simulink model "xNeuralSim_603"  (R2012b)
settings: Solver=FixedStepDiscrete  StartTime=0  StopTime=Inf  FixedStep=.0005  RelTol=1e-3
values from neighbouring files (symbols this model uses):
  cbhwlib_ver_major = 3    [buildXNeuralSim.m]    (also in xNeuralSim_Init.m)
  cbhwlib_ver_minor = 10    [buildXNeuralSim.m]    (also in xNeuralSim_Init.m = 9)
  enableNeuralSim = 1    [xNeuralSim_Init.m]
  max_num_cbpkts = 5    [xNeuralSim_Init.m]
  nch = 192    [xNeuralSim_Init.m]
  nsp_recv_port = 1001    [xNeuralSim_Init.m]
  nsp_send_port = 1002    [xNeuralSim_Init.m]
  sampleSendEnable_NSP1 = 1    [xNeuralSim_Init.m]
  sampleSendEnable_NSP2 = 1    [xNeuralSim_Init.m]
  spikeSendEnable_NSP1 = 1    [xNeuralSim_Init.m]
  spikeSendEnable_NSP2 = 1    [xNeuralSim_Init.m]
  unitMap = unitMap./repmat(sqrt(sum(unitMap.^2)), dimensions, 1)    [xNeuralSim_Init.m]
undefined symbols (not defined in the file or in its folder): macaddr
undefined symbols (not defined in the file): nsp1_pci_bus, nsp1_pci_slot
libraries: xpcethernetlib x15, xpcrtudplib x8, dspmtrx3 x7, xpclib x6, simulink x4, dspsrcs4 x2, xpciplib x2, xpcparallelportlib x1
(part 1 of 2)
settings Model: xpc_rtwmakecfg_data=_xpcetherlib__xpcether8255xlib__xpcetherGbElib__xpciplib__xpcnblib_  SimulationMode=external  TunableVars=enableNeuralSim  TunableVarsStorageClass=Auto  Creator=operator  LastModifiedBy=NPTL
settings SolverCC: EnableConcurrentExecution=on  InsertRTBMode=Always
settings DataIOCC: SignalLoggingSaveFormat=ModelDataLogs  DSMLogging=off
settings OptimizationCC: BlockReduction=off  InlineParams=on  InlineInvariantSignals=on  EnhancedBackFolding=on  EfficientFloat2IntCast=on  SimCompilerOptimization=On  AccelVerboseBuild=on
settings DebuggingCC: InheritedTsInSrcMsg=none  FcnCallInpInsideContextMsg=UseLocalSettings
settings HardwareCC: ProdIntDivRoundTo=Zero  ProdEndianess=LittleEndian  ProdHWDeviceType=Generic->32-bit x86 compatible
settings ModelReferenceCC: UpdateModelReferenceTargets=Force  EnableParallelModelReferenceBuilds=on
settings SFSimCC: SimBuildMode=sf_make_clean
settings RTWCC: SystemTargetFile=xpctarget.tlc  TLCOptions=-axPCMaxOverloads=100000  TemplateMakefile=xpc_default_tmf  Description=xPC Target  ProcessScript=xpctarget_make_rtw_hook  RTWCompilerOptimization=On
settings xpcTargetCC: TargetFcnLib=ansi_tfl_table_tmw.mat  CodeReplacementLibrary=XPC_BLAS  ParMdlRefBuildCompliant=on  ConcurrentExecutionCompliant=on  CombineSignalStateStructs=off  GRTInterface=on  RL32LogBufSizeModifier=10000  xPCTaskExecutionProfile=off  xPCRL32EventNumber=5000  RL32ObjectName=tgs  xPCisDefaultEnv=off  xPCTargetPCEnvName=xSimTarget  xPCLoadParamSetFile=off  xPCConcurrentTasks=on  xPCEnableSFAnimation=off

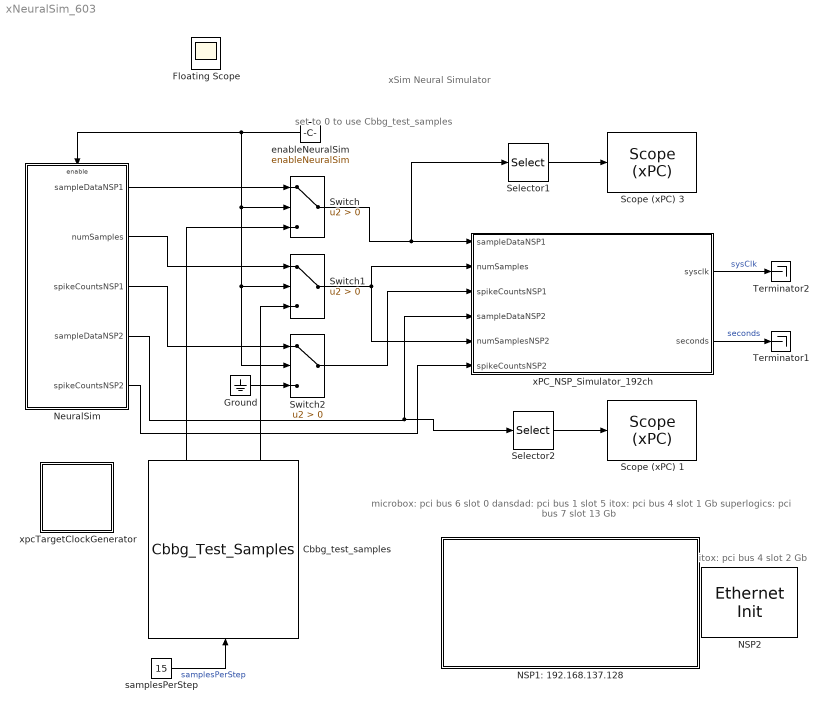
== system xNeuralSim_603 ==
  note: set to 0 to use
      | Cbbg_test_samples
  note: microbox: pci bus 6 slot 0
      | dansdad: pci bus 1 slot 5
      | itox: pci bus 4 slot 1 Gb
      | superlogics: pci bus 7 slot 13 Gb
  note: itox: pci bus 4 slot 2 Gb
  note: xSim Neural Simulator
  Cbbg_test_samples : S-Function  InitFcn=try, set_param(gcb,'FunctionName','Cbbg_Test_Samples'), end  FunctionName=Cbbg_Test_Samples  SFunctionModules=Cbbg_Test_Samples_wrapper  EnableBusSupport=off  mask(S-Function Builder){}
      mask help: The S-Function Builder block creates a wrapper C-MEX S-function from your supplied C code with multiple input ports, output ports, and a variable number of scalar, vector, or matrix parameters. The input and output ports can propagate Simulink built-in data types, fixed-point datatypes, complex, frame, 1-D, and 2-D signals. This block also supports discrete and continuous states of type real. You can optionally have the block generate a TLC file to be used with Real-Time Workshop for code generation.
      mask init:
      | val = [[.9  0.75 0.75 1 1 .9 .9 1]',[1 1 0.75 0.75 .9 .9 1 .9]'];try , sys = get_param(gcb,'SfunBuilderFcnName');if isempty(sys), sys = get_param(gcb,'FunctionName'); end,catch, sys = get_param(gcb,'FunctionName'); end
      settings: CopyFcn=set_param(gcbh,'LinkStatus','none')  PreSaveFcn=try, set_param(gcb,'FunctionName','Cbbg_Test_Samples'), end  OpenFcn=sfunctionwizard(gcbh)
      mask Display: plot(val(:,1),val(:,2)),disp(sys), port_label('input',1,'samplesPerStep'), port_label('output',1,'sampleData'), port_label('output',2,'numSamples')
  Ground : Ground
  NSP1: 192.168.137.128 : Subsystem  mask(xpcnwconfig){IpAddress=192.168.137.128, SubnetMask=255.255.255.0, Gateway=0.0.0.0, EthDrv=Intel Gigabit, PciBus=nsp1_pci_bus, PciSlot=nsp1_pci_slot}
      mask prompts: IpAddress "IP Address:"; SubnetMask "Subnet Mask:"; EthDrv "Ethernet Driver"; PciBus "PCI Bus:"; PciSlot "PCI Slot:"
      mask help: Network Configuration
      mask init:
      | IpAddress = ipaddr(IpAddress);
      | SubnetMask = ipaddr(SubnetMask);
      | Gateway = ipaddr(Gateway);
      mask Help: eval('xpcdoc(''RT_NETWORK_CONFIGURATION'')');
      mask TypeOptions EthDrv: Intel 8255x | Intel Gigabit
      mask Display: image(imread('cerebus.png','png'));
  NSP2 : xpcethernetlib/Ethernet Init   ID=2  Driver=Intel Gigabit  Bus=nsp2_pci_bus  Slot=nsp2_pci_slot  SampleTime=-1  AddressSource=EEPROM  MAC=macaddr('2A:2B:3C:4D:5E:6F')  TxSA=off  RxPromiscuous=off  Multicast={}  RxBad=off  RxShort=off  MaxMTU=1518  TxThreshold=224  TxBuffers=8192  RxBuffers=8192  ShowTune=on  NumRxBlks=1
  NeuralSim : Subsystem
  Scope (xPC) 1 : xpclib/Misc./Scope (xPC)   scopeno=4  scopetype=Target  autostart=on  viewmode=Graphical sliding  formatstr='%15.6f'  grid=on  ylimits=[-600 600]  nosamples=1000  noprepostsamples=0  interleave=1  triggermode=FreeRun  triggersignal=1  triggerlevel=-400  triggerslope=Falling  triggerscope=1  triggersample=0  filename=data.dat  mode=Lazy  writesize=512  autorestart=off  dynamicfilemode=off  maxwritefilesize=512*1024^2
  Scope (xPC) 3 : xpclib/Misc./Scope (xPC)   scopeno=3  scopetype=Target  autostart=on  viewmode=Graphical sliding  formatstr='%15.6f'  grid=on  ylimits=[-600 600]  nosamples=1000  noprepostsamples=0  interleave=1  triggermode=FreeRun  triggersignal=1  triggerlevel=-400  triggerslope=Falling  triggerscope=1  triggersample=0  filename=data.dat  mode=Lazy  writesize=512  autorestart=off  dynamicfilemode=off  maxwritefilesize=512*1024^2
  Selector1 : Selector  IndexOptions=Index vector (dialog)  Indices=[1440]  OutputSizes=1
  Selector2 : Selector  IndexOptions=Index vector (dialog)  Indices=[1440]  OutputSizes=1
  Switch : Switch  Criteria=u2 > Threshold
  Switch1 : Switch  Criteria=u2 > Threshold
  Switch2 : Switch  Criteria=u2 > Threshold
  Terminator1 : Terminator
  Terminator2 : Terminator
  enableNeuralSim : Constant  Value=enableNeuralSim  OutDataTypeStr=Inherit: Inherit via back propagation
  samplesPerStep : Constant  Value=15  OutDataTypeStr=Inherit: Inherit via back propagation
  xPC_NSP_Simulator_192ch : Subsystem
  xpcTargetClockGenerator : Subsystem
  Floating Scope : Scope
      settings: Floating=on
  wires:
  xPC_NSP_Simulator_192ch/2(seconds) -> Terminator1/1  "seconds"
  NeuralSim/1(sampleDataNSP1) -> Switch/1
  NeuralSim/2(numSamples) -> Switch1/1
  NeuralSim/3(spikeCountsNSP1) -> Switch2/1
  Cbbg_test_samples/1 -> Switch/3
  Switch1/1 -> xPC_NSP_Simulator_192ch/5(numSamplesNSP2), xPC_NSP_Simulator_192ch/2(numSamples)
  Cbbg_test_samples/2 -> Switch1/3
  enableNeuralSim/1 -> NeuralSim/Enable, Switch2/2, Switch1/2, Switch/2
  samplesPerStep/1 -> Cbbg_test_samples/1  "samplesPerStep"
  xPC_NSP_Simulator_192ch/1(sysclk) -> Terminator2/1  "sysClk"
  Selector1/1 -> Scope (xPC) 3/1
  Switch2/1 -> xPC_NSP_Simulator_192ch/3(spikeCountsNSP1)
  Ground/1 -> Switch2/3
  Switch/1 -> Selector1/1, xPC_NSP_Simulator_192ch/1(sampleDataNSP1)
  NeuralSim/5(spikeCountsNSP2) -> xPC_NSP_Simulator_192ch/6(spikeCountsNSP2)
  Selector2/1 -> Scope (xPC) 1/1
  NeuralSim/4(sampleDataNSP2) -> Selector2/1, xPC_NSP_Simulator_192ch/4(sampleDataNSP2)

== system xNeuralSim_603/NSP1: 192.168.137.128 ==
  "ARP Init " : S-Function  Priority=0  FunctionName=xpcdebugarpinit  Parameters=Stats, Interface, IpAddress, SubnetMask, Gateway, EthernetId, Flags, BlockId, Retry, Timeout, Expiration, StaticAddressListIp, StaticAddressListMac, DiscoveryList, MulticastList, SampleTime  EnableBusSupport=off  mask(arpinit){Interface=0, IpAddress=IpAddress, SubnetMask=SubnetMask, Gateway=Gateway, EthernetId=1, BlockId=0, SampleTime=-1, Flags=hex2dec('00000697'), Stats=off, Retry=5, Timeout=20, Expiration=20*60, StaticAddressListIp=[], StaticAddressListMac=[], DiscoveryList=[], MulticastList=[]}
      mask prompts: IpAddress "IP Address"; SubnetMask "Subnet Mask"; EthernetId "Ethernet ID"; BlockId "Block ID"; SampleTime "Sample Time"; Stats "Statistics Port"; StaticAddressListIp "[Static IP]"; StaticAddressListMac "[Static MAC]"; DiscoveryList "[Discovery IP]"; MulticastList "[Multicast IP]"
      mask help: ARP Init
      mask init:
      | xpclinklib('xpciplib');
      mask Help: web('arpdebug.htm',  '-helpbrowser');
      mask Display: disp('ARP Init');
  "Buffer Mngmt " : S-Function  Priority=-1  FunctionName=xpcnb  Parameters=pool_sizes, SampleTime, ShowTune  EnableBusSupport=off  mask(xpcnbinit){SampleTime=-1, PoolSizes=[2048 2048 50000 50000], ShowTune=on}
      mask prompts: SampleTime "Sample time:"; PoolSizes "Buffer pool sizes (256, 512, 1024, 2048):"; ShowTune "Display tuning information"
      mask help: Network Buffer Initialization
      mask init:
      | [MaskDisplay, pool_sizes] = mxpcnbinit(2, PoolSizes);
      | 
      | set_param(gcb, 'MaskDisplay', MaskDisplay);
      mask Help: eval('xpcdoc(''NB_Init'')');
      mask Display: disp('Network Buffer\nManagement');
  "Ethernet Init " : S-Function  Priority=-1  FunctionName=xpcetherinit  Parameters="ID, Driver, Bus, Slot, VendorID, DeviceID, AddressSource, mac, TxSA, RxPromiscuous, RxBad, RxShort, MaxMTU, TxThreshold, TxBuffers, RxBuffers, ShowTune, numMulti, multicast,   NumRxBlks, SampleTime"  EnableBusSupport=off  mask(xpcetherinit){ID=1, Driver=EthDrv, Bus=PciBus, Slot=PciSlot, SampleTime=-1, AddressSource=EEPROM, MAC=macaddr('00:00:00:00:00:00'), TxSA=off, RxPromiscuous=off, Multicast={}, RxBad=off, RxShort=off, MaxMTU=1518, TxThreshold=224, TxBuffers=8192, RxBuffers=8192, ShowTune=on, NumRxBlks=1}
      mask prompts: ID "Device ID:"; Bus "PCI bus:"; Slot "PCI slot:"; SampleTime "Sample time:"; AddressSource "Address source:"; TxSA "Tx source address from model"; RxPromiscuous "Rx promiscuous"; Multicast "Multicast address list:"; RxBad "Rx bad frames"; RxShort "Rx short frames"; MaxMTU "Max MTU:"; TxThreshold "Tx threshold:"; TxBuffers "Tx buffers:"; RxBuffers "Rx buffers:"; ShowTune "Display tuning information"; NumRxBlks "num rx blocks"
      mask help: Ethernet Initialization
      mask init:
      | VendorID = -1;
      | DeviceID = -1;
      | 
      | [MaskDisplay, VendorID, DeviceID, mac, numMulti, multicast] = mxpcetherinit(2, ID, Driver, Bus, Slot, MAC, Multicast);
      | 
      | set_param(gcb, 'MaskDisplay', MaskDisplay);
      mask Help: eval('xpcdoc(''Ether_Init'')');
      mask TypeOptions ID: 1 | 2 | 3 | 4 | 5 | 6 | 7 | 8
      mask TypeOptions AddressSource: EEPROM | Specify
      mask Callback AddressSource:
      | enables = get_param(gcb, 'MaskVisibilities');
      | if strcmp('Specify', get_param(gcb, 'AddressSource'))
      |     enables{strmatch('MAC',fieldnames(get_param(gcb,'DialogParameters')))} = 'on';
      | else
      |     enables{strmatch('MAC',fieldnames(get_param(gcb,'DialogParameters')))} = 'off';
      | end
      | set_param(gcb, 'MaskVisibilities', enables);
      mask Display: disp('Ethernet\nInitialization\nbus: 4 slot: 0\nId: 1\nIntel Gigabit');
  "IP Init " : S-Function  Priority=1  FunctionName=xpcdebugipinit  Parameters=Stats, Group, ArpId, IpAddress, SubnetMask, DefaultGateway, DefaultInterface, Flags, ToS, StartingId, TTL, SampleTime  EnableBusSupport=off  mask(ipinit){Group=0, ArpId=[0], IpAddress=[IpAddress], SubnetMask=[SubnetMask], DefaultGateway=Gateway, DefaultInterface=0, SampleTime=-1, Flags=hex2dec('00000005'), ToS=hex2dec('00'), StartingId=10000, TTL=64, Stats=off}
      mask prompts: ArpId "[ARP ID]"; IpAddress "[IP Address]"; SubnetMask "[Subnet Mask]"; DefaultGateway "Default Gateway"; DefaultInterface "Default Interface"; SampleTime "Sample Time"; StartingId "Starting Id"; Stats "Statistics Port"
      mask help: IP Init
      mask init:
      | xpclinklib('xpciplib');
      mask Help: web('ipdebug.htm',  '-helpbrowser');
      mask Display: disp('IP Init');
  "UDP Init " : S-Function  Priority=2  FunctionName=xpcdebugudpinit  Parameters=Stats, Group, StartingPort, Flags, SampleTime  EnableBusSupport=off  mask(udpinit){Group=0, StartingPort=10000, Flags=hex2dec('00000001'), SampleTime=-1, Stats=off}
      mask prompts: StartingPort "Starting Port"; SampleTime "Sample Time"; Stats "Statistics Port"
      mask help: UDP Init
      mask init:
      | xpclinklib('xpciplib');
      mask Help: web('udpdebug.htm',  '-helpbrowser');
      mask Display: disp('UDP Init');

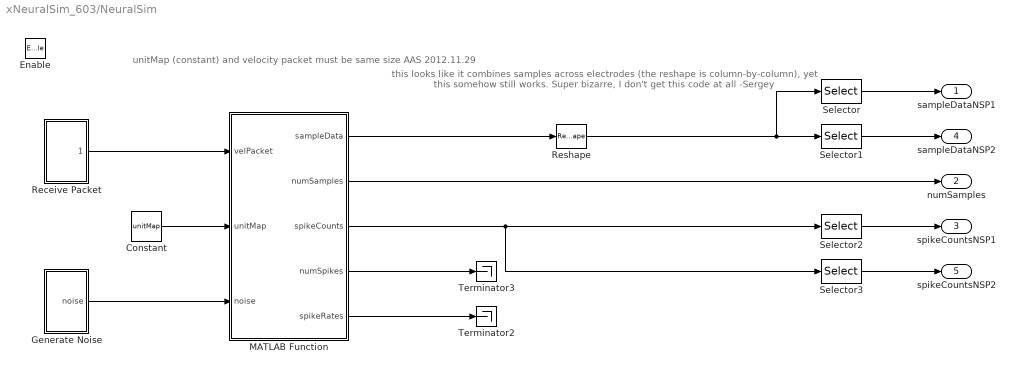
== system xNeuralSim_603/NeuralSim ==
  note: this looks like it combines samples across
      | electrodes (the reshape is column-by-column), yet this somehow still works.
      | Super bizarre, I don't get this code at all -Sergey
  note: unitMap (constant) and velocity
      | packet must be same size
      | AAS 2012.11.29
  Enable : EnablePort
  Constant : Constant  Value=unitMap
  Generate Noise : Subsystem
  MATLAB Function : MATLAB Function  TreatAsAtomicUnit=on
  Receive Packet : Subsystem
  Reshape : Reshape
  Selector : Selector  InputPortWidth=2880  IndexOptions=Starting index (dialog)  Indices=[1]  OutputSizes=1440
  Selector1 : Selector  InputPortWidth=2880  IndexOptions=Starting index (dialog)  Indices=[1441]  OutputSizes=1440
  Selector2 : Selector  InputPortWidth=192  IndexOptions=Starting index (dialog)  Indices=[1]  OutputSizes=96
  Selector3 : Selector  InputPortWidth=192  IndexOptions=Starting index (dialog)  Indices=[97]  OutputSizes=96
  Terminator2 : Terminator
  Terminator3 : Terminator
  sampleDataNSP1 : Outport
  numSamples : Outport  Port=2
  spikeCountsNSP1 : Outport  Port=3
  sampleDataNSP2 : Outport  Port=4
  spikeCountsNSP2 : Outport  Port=5
  wires:
  MATLAB Function/2(numSamples) -> numSamples/1
  MATLAB Function/4(numSpikes) -> Terminator3/1
  MATLAB Function/5(spikeRates) -> Terminator2/1
  Constant/1 -> MATLAB Function/2(unitMap)
  Receive Packet/1(velocity) -> MATLAB Function/1(velPacket)
  Generate Noise/1(noise) -> MATLAB Function/3(noise)
  Reshape/1 -> Selector/1, Selector1/1
  Selector/1 -> sampleDataNSP1/1
  Selector1/1 -> sampleDataNSP2/1
  Selector2/1 -> spikeCountsNSP1/1
  MATLAB Function/3(spikeCounts) -> Selector3/1, Selector2/1
  Selector3/1 -> spikeCountsNSP2/1
  MATLAB Function/1(sampleData) -> Reshape/1

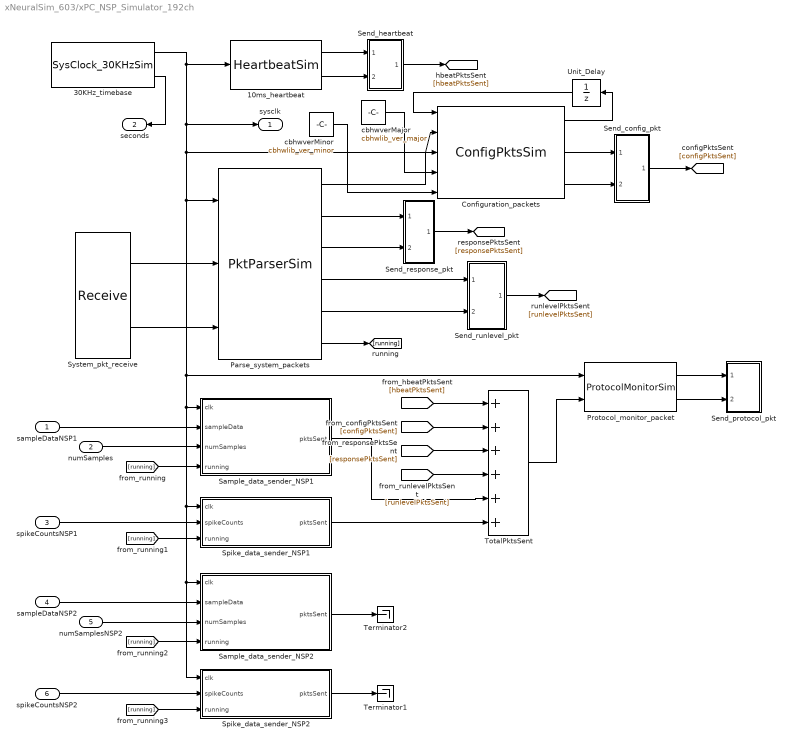
== system xNeuralSim_603/xPC_NSP_Simulator_192ch ==
  sampleDataNSP1 : Inport
  numSamples : Inport  Port=2
  spikeCountsNSP1 : Inport  Port=3
  sampleDataNSP2 : Inport  Port=4
  numSamplesNSP2 : Inport  Port=5
  spikeCountsNSP2 : Inport  Port=6
  10ms_heartbeat : S-Function  InitFcn=try, set_param(gcb,'FunctionName','HeartbeatSim'), end  FunctionName=HeartbeatSim  SFunctionModules=HeartbeatSim_wrapper  EnableBusSupport=off  mask(S-Function Builder){}
      mask help: The S-Function Builder block creates a wrapper C-MEX S-function from your supplied C code with multiple input ports, output ports, and a variable number of scalar, vector, or matrix parameters. The input and output ports can propagate Simulink built-in data types, fixed-point datatypes, complex, frame, 1-D, and 2-D signals. This block also supports discrete and continuous states of type real. You can optionally have the block generate a TLC file to be used with Real-Time Workshop for code generation.
      mask init: same as xNeuralSim_603/Cbbg_test_samples
      settings: CopyFcn=set_param(gcbh,'LinkStatus','none')  PreSaveFcn=try, set_param(gcb,'FunctionName','HeartbeatSim'), end  OpenFcn=sfunctionwizard(gcbh)
      mask Display: plot(val(:,1),val(:,2)),disp(sys), port_label('input',1,'clk'), port_label('output',1,'pktData'), port_label('output',2,'pktSize')
  30KHz_timebase : S-Function  InitFcn=try, set_param(gcb,'FunctionName','SysClock_30KHzSim'), end  FunctionName=SysClock_30KHzSim  SFunctionModules=SysClock_30KHzSim_wrapper  EnableBusSupport=off  mask(S-Function Builder){}
      mask help: The S-Function Builder block creates a wrapper C-MEX S-function from your supplied C code with multiple input ports, output ports, and a variable number of scalar, vector, or matrix parameters. The input and output ports can propagate Simulink built-in data types, fixed-point datatypes, complex, frame, 1-D, and 2-D signals. This block also supports discrete and continuous states of type real. You can optionally have the block generate a TLC file to be used with Real-Time Workshop for code generation.
      mask init: same as xNeuralSim_603/Cbbg_test_samples
      settings: CopyFcn=set_param(gcbh,'LinkStatus','none')  PreSaveFcn=try, set_param(gcb,'FunctionName','SysClock_30KHzSim'), end  OpenFcn=sfunctionwizard(gcbh)
      mask Display: plot(val(:,1),val(:,2)),disp(sys), port_label('output',1,'clk'), port_label('output',2,'seconds')
  Configuration_packets : S-Function  InitFcn=try, set_param(gcb,'FunctionName','ConfigPktsSim'), end  FunctionName=ConfigPktsSim  SFunctionModules=ConfigPktsSim_wrapper  EnableBusSupport=off  mask(S-Function Builder){}
      mask help: The S-Function Builder block creates a wrapper C-MEX S-function from your supplied C code with multiple input ports, output ports, and a variable number of scalar, vector, or matrix parameters. The input and output ports can propagate Simulink built-in data types, fixed-point datatypes, complex, frame, 1-D, and 2-D signals. This block also supports discrete and continuous states of type real. You can optionally have the block generate a TLC file to be used with Real-Time Workshop for code generation.
      mask init: same as xNeuralSim_603/Cbbg_test_samples
      settings: CopyFcn=set_param(gcbh,'LinkStatus','none')  PreSaveFcn=try, set_param(gcb,'FunctionName','ConfigPktsSim'), end  OpenFcn=sfunctionwizard(gcbh)
      mask Display: plot(val(:,1),val(:,2)),disp(sys), port_label('input',1,'continue_in'), port_label('input',2,'clk'), port_label('input',3,'start'), port_label('input',4,'cbhwverMajor'), port_label('input',5,'cbhwverMinor'), port_label('output',1,'continue_out'), port_label('output',2,'pktData'), port_label('output',3,'pktSize')
  Parse_system_packets : S-Function  InitFcn=try, set_param(gcb,'FunctionName','PktParserSim'), end  FunctionName=PktParserSim  SFunctionModules=PktParserSim_wrapper  EnableBusSupport=off  mask(S-Function Builder){}
      mask help: The S-Function Builder block creates a wrapper C-MEX S-function from your supplied C code with multiple input ports, output ports, and a variable number of scalar, vector, or matrix parameters. The input and output ports can propagate Simulink built-in data types, fixed-point datatypes, complex, frame, 1-D, and 2-D signals. This block also supports discrete and continuous states of type real. You can optionally have the block generate a TLC file to be used with Real-Time Workshop for code generation.
      mask init: same as xNeuralSim_603/Cbbg_test_samples
      settings: CopyFcn=set_param(gcbh,'LinkStatus','none')  PreSaveFcn=try, set_param(gcb,'FunctionName','PktParserSim'), end  OpenFcn=sfunctionwizard(gcbh)
      mask Display: plot(val(:,1),val(:,2)),disp(sys), port_label('input',1,'clk'), port_label('input',2,'data'), port_label('input',3,'size'), port_label('output',1,'sendConfigPkts'), port_label('output',2,'responsePktData'), port_label('output',3,'responsePktSize'), port_label('output',4,'setRunlevelPktData'), port_label('output',5,'setRunlevelPktSize'), port_label('output',6,'running')
  Protocol_monitor_packet : S-Function  InitFcn=try, set_param(gcb,'FunctionName','ProtocolMonitorSim'), end  FunctionName=ProtocolMonitorSim  SFunctionModules=ProtocolMonitorSim_wrapper  EnableBusSupport=off  mask(S-Function Builder){}
      mask help: The S-Function Builder block creates a wrapper C-MEX S-function from your supplied C code with multiple input ports, output ports, and a variable number of scalar, vector, or matrix parameters. The input and output ports can propagate Simulink built-in data types, fixed-point datatypes, complex, frame, 1-D, and 2-D signals. This block also supports discrete and continuous states of type real. You can optionally have the block generate a TLC file to be used with Real-Time Workshop for code generation.
      mask init: same as xNeuralSim_603/Cbbg_test_samples
      settings: CopyFcn=set_param(gcbh,'LinkStatus','none')  PreSaveFcn=try, set_param(gcb,'FunctionName','ProtocolMonitorSim'), end  OpenFcn=sfunctionwizard(gcbh)
      mask Display: plot(val(:,1),val(:,2)),disp(sys), port_label('input',1,'clk'), port_label('input',2,'pktsSent'), port_label('output',1,'pktData'), port_label('output',2,'pktSize')
  Sample_data_sender_NSP1 : Subsystem  TreatAsAtomicUnit=on
  Sample_data_sender_NSP2 : Subsystem  TreatAsAtomicUnit=on
  Send_config_pkt : Subsystem
  Send_heartbeat : Subsystem
  Send_protocol_pkt : Subsystem
  Send_response_pkt : Subsystem
  Send_runlevel_pkt : Subsystem
  Spike_data_sender_NSP1 : Subsystem  TreatAsAtomicUnit=on
  Spike_data_sender_NSP2 : Subsystem  TreatAsAtomicUnit=on
  "System_pkt_receive " : xpcrtudplib/Receive   Receive1=0.0.0.0  Receive2=nsp_recv_port  Receive3=1024*16  Receive4=-1
  Terminator1 : Terminator
  Terminator2 : Terminator
  TotalPktsSent : Sum  Inputs=++++++
  Unit_Delay : UnitDelay  SampleTime=-1
  cbhwverMajor : Constant  Value=cbhwlib_ver_major  OutDataTypeStr=uint16
  cbhwverMinor : Constant  Value=cbhwlib_ver_minor  OutDataTypeStr=uint16
  sysclk : Outport
  seconds : Outport  Port=2
  wires:
  30KHz_timebase/1 -> 10ms_heartbeat/1, Configuration_packets/2, Spike_data_sender_NSP1/1(clk), Spike_data_sender_NSP2/1(clk), Sample_data_sender_NSP2/1(clk), Sample_data_sender_NSP1/1(clk), Protocol_monitor_packet/1, Parse_system_packets/1, sysclk/1
  "System_pkt_receive "/1 -> Parse_system_packets/2
  Unit_Delay/1 -> Configuration_packets/1
  Configuration_packets/2 -> Send_config_pkt/1(pktData)
  Configuration_packets/3 -> Send_config_pkt/2(pktSize)
  10ms_heartbeat/1 -> Send_heartbeat/1(pktData)
  10ms_heartbeat/2 -> Send_heartbeat/2(pktSize)
  Parse_system_packets/2 -> Send_response_pkt/1(pktData)
  Parse_system_packets/3 -> Send_response_pkt/2(pktSize)
  Protocol_monitor_packet/1 -> Send_protocol_pkt/1(pktData)
  Protocol_monitor_packet/2 -> Send_protocol_pkt/2(pktSize)
  Parse_system_packets/1 -> Configuration_packets/3
  "System_pkt_receive "/2 -> Parse_system_packets/3
  sampleDataNSP1/1 -> Sample_data_sender_NSP1/2(sampleData)
  Send_heartbeat/1(pktsSent) -> [hbeatPktsSent]
  Parse_system_packets/4 -> Send_runlevel_pkt/1(pktData)
  Parse_system_packets/5 -> Send_runlevel_pkt/2(pktSize)
  Parse_system_packets/6 -> [running]
  Send_response_pkt/1(pktsSent) -> [responsePktsSent]
  Send_runlevel_pkt/1(pktsSent) -> [runlevelPktsSent]
  [hbeatPktsSent] -> TotalPktsSent/1
  [configPktsSent] -> TotalPktsSent/2
  [responsePktsSent] -> TotalPktsSent/3
  [runlevelPktsSent] -> TotalPktsSent/4
  Sample_data_sender_NSP1/1(pktsSent) -> TotalPktsSent/5
  Send_config_pkt/1(pktsSent) -> [configPktsSent]
  Configuration_packets/1 -> Unit_Delay/1
  30KHz_timebase/2 -> seconds/1
  [running] -> Sample_data_sender_NSP1/4(running)
  numSamples/1 -> Sample_data_sender_NSP1/3(numSamples)
  spikeCountsNSP1/1 -> Spike_data_sender_NSP1/2(spikeCounts)
  [running] -> Spike_data_sender_NSP1/3(running)
  TotalPktsSent/1 -> Protocol_monitor_packet/2
  Spike_data_sender_NSP1/1(pktsSent) -> TotalPktsSent/6
  sampleDataNSP2/1 -> Sample_data_sender_NSP2/2(sampleData)
  [running] -> Sample_data_sender_NSP2/4(running)
  numSamplesNSP2/1 -> Sample_data_sender_NSP2/3(numSamples)
  spikeCountsNSP2/1 -> Spike_data_sender_NSP2/2(spikeCounts)
  [running] -> Spike_data_sender_NSP2/3(running)
  Sample_data_sender_NSP2/1(pktsSent) -> Terminator2/1
  Spike_data_sender_NSP2/1(pktsSent) -> Terminator1/1
  cbhwverMajor/1 -> Configuration_packets/4
  cbhwverMinor/1 -> Configuration_packets/5

== system xNeuralSim_603/xpcTargetClockGenerator ==
  "Parallel Port DO " : xpcparallelportlib/Digital Output/Parallel Port DO   BaseMask=0x378  BaseString=0x378  Format=8 1-bit Channels  Channels=[1]  InitialValues=[0]  FinalActions=[0]  FinalValues=[0]  SampleTime=-1  Mode=1
  cerebus Parallel : MATLAB Function  TreatAsAtomicUnit=on
  wires:
  cerebus Parallel/1(digitalOut) -> "Parallel Port DO "/1

== system xNeuralSim_603/NeuralSim/Generate Noise ==
  Data Type  Conversion : DataTypeConversion  OutDataTypeStr=int16  RndMeth=Zero
  Random Source : dspsrcs4/Random Source  SrcType=Gaussian  NormMethod=Ziggurat  CltLength=12  MinVal=0  MaxVal=1  MeanVal=0  VarVal=noiseScaleFactor  RepMode=Specify seed  rawSeed=1  IsInherit=off  SampMode=Discrete  SampTime=-1  SampFrame=nch*15  DataType=Double  OutComplex=Real
  Random Source1 : dspsrcs4/Random Source  SrcType=Uniform  NormMethod=Ziggurat  CltLength=12  MinVal=0  MaxVal=noiseScaleFactor  MeanVal=0  VarVal=noiseScaleFactor  RepMode=Specify seed  rawSeed=1  IsInherit=off  SampMode=Discrete  SampTime=-1  SampFrame=nch*15  DataType=Double  OutComplex=Real
  Reshape1 : Reshape  OutputDimensionality=Customize  OutputDimensions=[nch,15]
  Reshape2 : Reshape  OutputDimensionality=Customize  OutputDimensions=[nch,15]
  Sum : Sum
  noise : Outport
  wires:
  Data Type  Conversion/1 -> noise/1
  Sum/1 -> Data Type  Conversion/1
  Reshape1/1 -> Sum/1
  Random Source/1 -> Reshape1/1
  Reshape2/1 -> Sum/2
  Random Source1/1 -> Reshape2/1

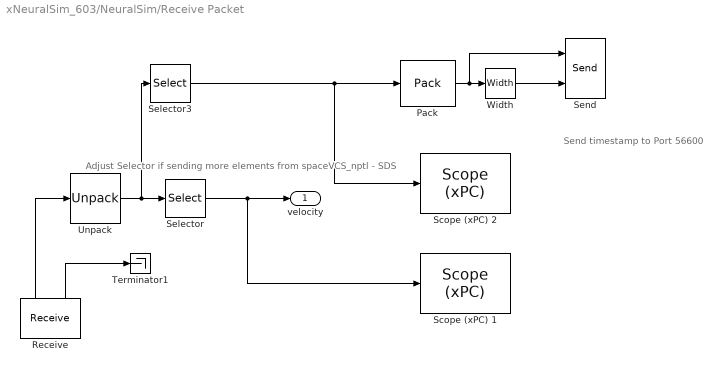
== system xNeuralSim_603/NeuralSim/Receive Packet ==
  note: Adjust Selector if sending more elements
      | from spaceVCS_nptl - SDS
  note: Send timestamp to Port 56600
  Pack : xpclib/UDP/Pack  datatypes={'double'}  byteAlign=1
  "Receive " : xpcrtudplib/Receive   Receive1=0.0.0.0  Receive2=49255  Receive3=8*64  Receive4=-1
  Scope (xPC) 1 : xpclib/Misc./Scope (xPC)   scopeno=1  scopetype=Target  autostart=on  viewmode=Numerical  formatstr='%15.6f'  grid=on  ylimits=[0,0]  nosamples=250  noprepostsamples=0  interleave=1  triggermode=FreeRun  triggersignal=1  triggerlevel=0.0  triggerslope=Either  triggerscope=1  triggersample=0  filename=data.dat  mode=Lazy  writesize=512  autorestart=off  dynamicfilemode=off  maxwritefilesize=512*1024^2
  Scope (xPC) 2 : xpclib/Misc./Scope (xPC)   scopeno=2  scopetype=Target  autostart=on  viewmode=Numerical  formatstr='%15.6f'  grid=on  ylimits=[0,0]  nosamples=250  noprepostsamples=0  interleave=1  triggermode=FreeRun  triggersignal=1  triggerlevel=0.0  triggerslope=Either  triggerscope=1  triggersample=0  filename=data.dat  mode=Lazy  writesize=512  autorestart=off  dynamicfilemode=off  maxwritefilesize=512*1024^2
  Selector : Selector  IndexOptions=Index vector (dialog)  Indices=[2 3 4 5 6 7]  OutputSizes=1
  Selector3 : Selector  IndexOptions=Index vector (dialog)  Indices=1  OutputSizes=1
  "Send " : xpcrtudplib/Send   Send1=192.168.137.255  Send2=56600  Send3=-1  Send4=-1
  Terminator1 : Terminator
  Unpack : xpclib/UDP/Unpack  dimensions={[64]}  datatypes={'double'}  byteAlign=1
  Width : Width
  velocity : Outport
  wires:
  Unpack/1 -> Selector3/1, Selector/1
  Width/1 -> "Send "/2
  Selector/1 -> Scope (xPC) 1/1, velocity/1
  Pack/1 -> "Send "/1, Width/1
  "Receive "/2 -> Terminator1/1
  "Receive "/1 -> Unpack/1
  Selector3/1 -> Scope (xPC) 2/1, Pack/1

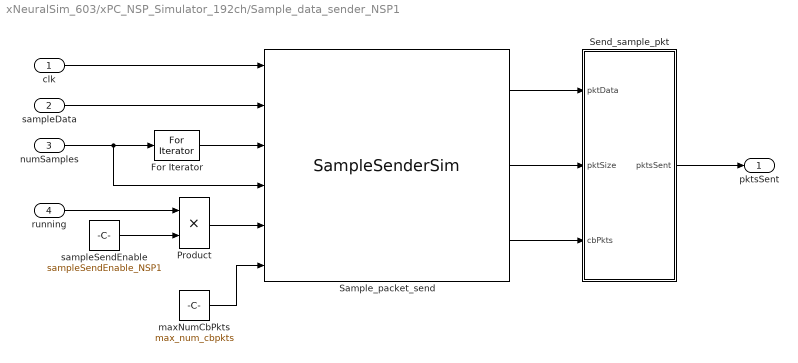
== system xNeuralSim_603/xPC_NSP_Simulator_192ch/Sample_data_sender_NSP1 ==
  clk : Inport
  sampleData : Inport  Port=2
  numSamples : Inport  Port=3
  running : Inport  Port=4
  For Iterator : ForIterator  IterationSource=external  IndexMode=Zero-based
  Product : Product  OutDataTypeStr=int32  RndMeth=Zero
  Sample_packet_send : S-Function  InitFcn=try, set_param(gcb,'FunctionName','SampleSenderSim'), end  FunctionName=SampleSenderSim  SFunctionModules=SampleSenderSim_wrapper  EnableBusSupport=off  mask(S-Function Builder){}
      mask help: The S-Function Builder block creates a wrapper C-MEX S-function from your supplied C code with multiple input ports, output ports, and a variable number of scalar, vector, or matrix parameters. The input and output ports can propagate Simulink built-in data types, fixed-point datatypes, complex, frame, 1-D, and 2-D signals. This block also supports discrete and continuous states of type real. You can optionally have the block generate a TLC file to be used with Real-Time Workshop for code generation.
      mask init: same as xNeuralSim_603/Cbbg_test_samples
      settings: CopyFcn=set_param(gcbh,'LinkStatus','none')  PreSaveFcn=try, set_param(gcb,'FunctionName','SampleSenderSim'), end  OpenFcn=sfunctionwizard(gcbh)
      mask Display: plot(val(:,1),val(:,2)),disp(sys), port_label('input',1,'clk'), port_label('input',2,'sampleData'), port_label('input',3,'sampleNum'), port_label('input',4,'numSamples'), port_label('input',5,'running'), port_label('input',6,'maxNumCbPkts'), port_label('output',1,'udpData'), port_label('output',2,'udpSize'), port_label('output',3,'cbPkts')
  Send_sample_pkt : Subsystem
  maxNumCbPkts : Constant  Value=max_num_cbpkts  OutDataTypeStr=int32
  sampleSendEnable : Constant  Value=sampleSendEnable_NSP1  OutDataTypeStr=int32
  pktsSent : Outport
  wires:
  For Iterator/1 -> Sample_packet_send/3
  sampleData/1 -> Sample_packet_send/2
  clk/1 -> Sample_packet_send/1
  numSamples/1 -> Sample_packet_send/4, For Iterator/1
  Send_sample_pkt/1(pktsSent) -> pktsSent/1
  Sample_packet_send/1 -> Send_sample_pkt/1(pktData)
  Sample_packet_send/2 -> Send_sample_pkt/2(pktSize)
  Sample_packet_send/3 -> Send_sample_pkt/3(cbPkts)
  running/1 -> Product/1
  sampleSendEnable/1 -> Product/2
  Product/1 -> Sample_packet_send/5
  maxNumCbPkts/1 -> Sample_packet_send/6

== system xNeuralSim_603/xPC_NSP_Simulator_192ch/Sample_data_sender_NSP2 ==
  clk : Inport
  sampleData : Inport  Port=2
  numSamples : Inport  Port=3
  running : Inport  Port=4
  For Iterator : ForIterator  IterationSource=external  IndexMode=Zero-based
  Product : Product  OutDataTypeStr=int32  RndMeth=Zero
  Sample_packet_send_NSP2 : S-Function  InitFcn=try, set_param(gcb,'FunctionName','SampleSenderSimNSP2'), end  FunctionName=SampleSenderSimNSP2  SFunctionModules=SampleSenderSimNSP2_wrapper  EnableBusSupport=off  mask(S-Function Builder){}
      mask help: The S-Function Builder block creates a wrapper C-MEX S-function from your supplied C code with multiple input ports, output ports, and a variable number of scalar, vector, or matrix parameters. The input and output ports can propagate Simulink built-in data types, fixed-point datatypes, complex, frame, 1-D, and 2-D signals. This block also supports discrete and continuous states of type real. You can optionally have the block generate a TLC file to be used with Real-Time Workshop for code generation.
      mask init: same as xNeuralSim_603/Cbbg_test_samples
      settings: CopyFcn=set_param(gcbh,'LinkStatus','none')  PreSaveFcn=try, set_param(gcb,'FunctionName','SampleSenderSimNSP2'), end  OpenFcn=sfunctionwizard(gcbh)
      mask Display: plot(val(:,1),val(:,2)),disp(sys), port_label('input',1,'clk'), port_label('input',2,'sampleData'), port_label('input',3,'sampleNum'), port_label('input',4,'numSamples'), port_label('input',5,'running'), port_label('input',6,'maxNumCbPkts'), port_label('output',1,'udpData'), port_label('output',2,'udpSize'), port_label('output',3,'cbPkts')
  Send_sample_pkt : Subsystem
  maxNumCbPkts : Constant  Value=max_num_cbpkts  OutDataTypeStr=int32
  sampleSendEnable : Constant  Value=sampleSendEnable_NSP2  OutDataTypeStr=int32
  pktsSent : Outport
  wires:
  For Iterator/1 -> Sample_packet_send_NSP2/3
  sampleData/1 -> Sample_packet_send_NSP2/2
  clk/1 -> Sample_packet_send_NSP2/1
  numSamples/1 -> Sample_packet_send_NSP2/4, For Iterator/1
  Send_sample_pkt/1(pktsSent) -> pktsSent/1
  Sample_packet_send_NSP2/1 -> Send_sample_pkt/1(pktData)
  Sample_packet_send_NSP2/2 -> Send_sample_pkt/2(pktSize)
  Sample_packet_send_NSP2/3 -> Send_sample_pkt/3(cbPkts)
  running/1 -> Product/1
  sampleSendEnable/1 -> Product/2
  Product/1 -> Sample_packet_send_NSP2/5
  maxNumCbPkts/1 -> Sample_packet_send_NSP2/6

== system xNeuralSim_603/xPC_NSP_Simulator_192ch/Send_config_pkt ==
  pktData : Inport
  pktSize : Inport  Port=2
  If : If  ShowElse=off
  If Action Subsystem : Subsystem  TreatAsAtomicUnit=on
  pktsSent : Outport
  wires:
  pktData/1 -> If Action Subsystem/1(pktData)
  If/1 -> If Action Subsystem/Action
  pktSize/1 -> If/1, If Action Subsystem/2(pktSize)
  If Action Subsystem/1(pktsSent) -> pktsSent/1

== system xNeuralSim_603/xPC_NSP_Simulator_192ch/Send_heartbeat ==
  pktData : Inport
  pktSize : Inport  Port=2
  If : If  ShowElse=off
  If Action Subsystem : Subsystem  TreatAsAtomicUnit=on
  pktsSent : Outport
  wires:
  pktData/1 -> If Action Subsystem/1(pktData)
  If/1 -> If Action Subsystem/Action
  pktSize/1 -> If/1, If Action Subsystem/2(pktSize)
  If Action Subsystem/1(pktsSent) -> pktsSent/1

== system xNeuralSim_603/xPC_NSP_Simulator_192ch/Send_protocol_pkt ==
  pktData : Inport
  pktSize : Inport  Port=2
  If : If  ShowElse=off
  If Action Subsystem : Subsystem  TreatAsAtomicUnit=on
  wires:
  pktData/1 -> If Action Subsystem/1(pktData)
  If/1 -> If Action Subsystem/Action
  pktSize/1 -> If/1, If Action Subsystem/2(pktSize)

== system xNeuralSim_603/xPC_NSP_Simulator_192ch/Send_response_pkt ==
  pktData : Inport
  pktSize : Inport  Port=2
  If : If  ShowElse=off
  If Action Subsystem : Subsystem  TreatAsAtomicUnit=on
  pktsSent : Outport
  wires:
  pktData/1 -> If Action Subsystem/1(pktData)
  If/1 -> If Action Subsystem/Action
  pktSize/1 -> If/1, If Action Subsystem/2(pktSize)
  If Action Subsystem/1(pktsSent) -> pktsSent/1

== system xNeuralSim_603/xPC_NSP_Simulator_192ch/Send_runlevel_pkt ==
  pktData : Inport
  pktSize : Inport  Port=2
  If : If  ShowElse=off
  If Action Subsystem : Subsystem  TreatAsAtomicUnit=on
  pktsSent : Outport
  wires:
  pktData/1 -> If Action Subsystem/1(pktData)
  If/1 -> If Action Subsystem/Action
  pktSize/1 -> If/1, If Action Subsystem/2(pktSize)
  If Action Subsystem/1(pktsSent) -> pktsSent/1

== system xNeuralSim_603/xPC_NSP_Simulator_192ch/Spike_data_sender_NSP1 ==
  clk : Inport
  spikeCounts : Inport  Port=2
  running : Inport  Port=3
  For Iterator : ForIterator  IterationSource=external  IndexMode=Zero-based
  Product : Product  OutDataTypeStr=int32  RndMeth=Zero
  Send_sample_pkt : Subsystem
  Spike_packet_send : S-Function  InitFcn=try, set_param(gcb,'FunctionName','SpikeSenderSim'), end  FunctionName=SpikeSenderSim  SFunctionModules=SpikeSenderSim_wrapper  EnableBusSupport=off  mask(S-Function Builder){}
      mask help: The S-Function Builder block creates a wrapper C-MEX S-function from your supplied C code with multiple input ports, output ports, and a variable number of scalar, vector, or matrix parameters. The input and output ports can propagate Simulink built-in data types, fixed-point datatypes, complex, frame, 1-D, and 2-D signals. This block also supports discrete and continuous states of type real. You can optionally have the block generate a TLC file to be used with Real-Time Workshop for code generation.
      mask init: same as xNeuralSim_603/Cbbg_test_samples
      settings: CopyFcn=set_param(gcbh,'LinkStatus','none')  PreSaveFcn=try, set_param(gcb,'FunctionName','SpikeSenderSim'), end  OpenFcn=sfunctionwizard(gcbh)
      mask Display: plot(val(:,1),val(:,2)),disp(sys), port_label('input',1,'clk'), port_label('input',2,'spikeCounts'), port_label('input',3,'chanNum'), port_label('input',4,'numChans'), port_label('input',5,'running'), port_label('output',1,'udpData'), port_label('output',2,'udpSize'), port_label('output',3,'cbPkts')
  Width : Width  DataType=int32
  spikeSendEnable : Constant  Value=spikeSendEnable_NSP1  OutDataTypeStr=int32
  pktsSent : Outport
  wires:
  For Iterator/1 -> Spike_packet_send/3
  spikeCounts/1 -> Width/1, Spike_packet_send/2
  clk/1 -> Spike_packet_send/1
  Send_sample_pkt/1(pktsSent) -> pktsSent/1
  Spike_packet_send/1 -> Send_sample_pkt/1(pktData)
  Spike_packet_send/2 -> Send_sample_pkt/2(pktSize)
  Spike_packet_send/3 -> Send_sample_pkt/3(cbPkts)
  Width/1 -> Spike_packet_send/4, For Iterator/1
  Product/1 -> Spike_packet_send/5
  running/1 -> Product/1
  spikeSendEnable/1 -> Product/2

== system xNeuralSim_603/xPC_NSP_Simulator_192ch/Spike_data_sender_NSP2 ==
  clk : Inport
  spikeCounts : Inport  Port=2
  running : Inport  Port=3
  For Iterator : ForIterator  IterationSource=external  IndexMode=Zero-based
  Product : Product  OutDataTypeStr=int32  RndMeth=Zero
  Send_sample_pkt : Subsystem
  Spike_packet_send_NSP2 : S-Function  InitFcn=try, set_param(gcb,'FunctionName','SpikeSenderSimNSP2'), end  FunctionName=SpikeSenderSimNSP2  SFunctionModules=SpikeSenderSimNSP2_wrapper  EnableBusSupport=off  mask(S-Function Builder){}
      mask help: The S-Function Builder block creates a wrapper C-MEX S-function from your supplied C code with multiple input ports, output ports, and a variable number of scalar, vector, or matrix parameters. The input and output ports can propagate Simulink built-in data types, fixed-point datatypes, complex, frame, 1-D, and 2-D signals. This block also supports discrete and continuous states of type real. You can optionally have the block generate a TLC file to be used with Real-Time Workshop for code generation.
      mask init: same as xNeuralSim_603/Cbbg_test_samples
      settings: CopyFcn=set_param(gcbh,'LinkStatus','none')  PreSaveFcn=try, set_param(gcb,'FunctionName','SpikeSenderSimNSP2'), end  OpenFcn=sfunctionwizard(gcbh)
      mask Display: plot(val(:,1),val(:,2)),disp(sys), port_label('input',1,'clk'), port_label('input',2,'spikeCounts'), port_label('input',3,'chanNum'), port_label('input',4,'numChans'), port_label('input',5,'running'), port_label('output',1,'udpData'), port_label('output',2,'udpSize'), port_label('output',3,'cbPkts')
  Width : Width  DataType=int32
  spikeSendEnable : Constant  Value=spikeSendEnable_NSP2  OutDataTypeStr=int32
  pktsSent : Outport
  wires:
  For Iterator/1 -> Spike_packet_send_NSP2/3
  spikeCounts/1 -> Width/1, Spike_packet_send_NSP2/2
  clk/1 -> Spike_packet_send_NSP2/1
  Send_sample_pkt/1(pktsSent) -> pktsSent/1
  Spike_packet_send_NSP2/1 -> Send_sample_pkt/1(pktData)
  Spike_packet_send_NSP2/2 -> Send_sample_pkt/2(pktSize)
  Spike_packet_send_NSP2/3 -> Send_sample_pkt/3(cbPkts)
  Width/1 -> Spike_packet_send_NSP2/4, For Iterator/1
  Product/1 -> Spike_packet_send_NSP2/5
  running/1 -> Product/1
  spikeSendEnable/1 -> Product/2

== system xNeuralSim_603/xPC_NSP_Simulator_192ch/Sample_data_sender_NSP1/Send_sample_pkt ==
  pktData : Inport
  pktSize : Inport  Port=2
  cbPkts : Inport  Port=3
  If : If  ShowElse=off
  If Action Subsystem : Subsystem  TreatAsAtomicUnit=on
  pktsSent : Outport
  wires:
  pktData/1 -> If Action Subsystem/1(pktData)
  If/1 -> If Action Subsystem/Action
  pktSize/1 -> If Action Subsystem/2(pktSize), If/1
  If Action Subsystem/1(pktsSent1) -> pktsSent/1
  cbPkts/1 -> If Action Subsystem/3(cbPkts1)

== system xNeuralSim_603/xPC_NSP_Simulator_192ch/Sample_data_sender_NSP2/Send_sample_pkt ==
  pktData : Inport
  pktSize : Inport  Port=2
  cbPkts : Inport  Port=3
  If : If  ShowElse=off
  If Action Subsystem : Subsystem  TreatAsAtomicUnit=on
  pktsSent : Outport
  wires:
  pktData/1 -> If Action Subsystem/1(pktData)
  If/1 -> If Action Subsystem/Action
  pktSize/1 -> If Action Subsystem/2(pktSize), If/1
  If Action Subsystem/1(pktsSent1) -> pktsSent/1
  cbPkts/1 -> If Action Subsystem/3(cbPkts1)

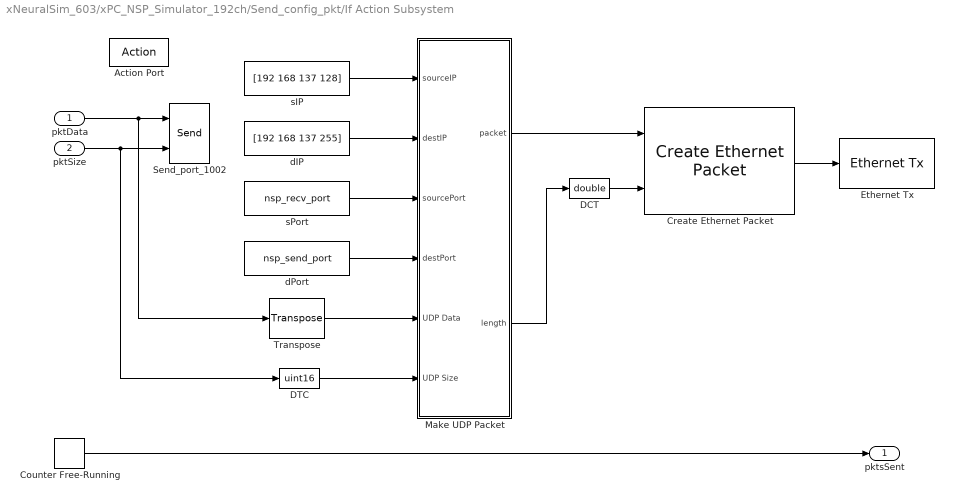
== system xNeuralSim_603/xPC_NSP_Simulator_192ch/Send_config_pkt/If Action Subsystem ==
  pktData : Inport
  pktSize : Inport  Port=2
  Action Port : ActionPort  ActionType=then
  Counter Free-Running : simulink/Sources/Counter Free-Running  NumBits=32  tsamp=-1
  Create Ethernet Packet : xpcethernetlib/Create Ethernet Packet   DstMac=macaddr('ff:ff:ff:ff:ff:ff')  EtherType=hex2dec('0800')
  DCT : DataTypeConversion  OutDataTypeStr=double
  DTC : DataTypeConversion  OutDataTypeStr=uint16
  Ethernet Tx : xpcethernetlib/Ethernet Tx   ID=2  SampleTime=-1
  Make UDP Packet : Subsystem
  Send_port_1002 : xpcrtudplib/Send   Send1=192.168.137.255  Send2=nsp_send_port  Send3=nsp_recv_port  Send4=-1
  Transpose : dspmtrx3/Transpose  Hermitian=off  overflowFlag=off
  dIP : Constant  Value=[192 168 137 255]  OutDataTypeStr=uint8
  dPort : Constant  Value=nsp_send_port  OutDataTypeStr=uint16
  sIP : Constant  Value=[192 168 137 128]  OutDataTypeStr=uint8
  sPort : Constant  Value=nsp_recv_port  OutDataTypeStr=uint16
  pktsSent : Outport  InitialOutput=0
  wires:
  Counter Free-Running/1 -> pktsSent/1
  DTC/1 -> Make UDP Packet/6(UDP Size)
  Make UDP Packet/2(length) -> DCT/1
  DCT/1 -> Create Ethernet Packet/2
  Make UDP Packet/1(packet) -> Create Ethernet Packet/1
  sPort/1 -> Make UDP Packet/3(sourcePort)
  Create Ethernet Packet/1 -> Ethernet Tx/1
  sIP/1 -> Make UDP Packet/1(sourceIP)
  dIP/1 -> Make UDP Packet/2(destIP)
  dPort/1 -> Make UDP Packet/4(destPort)
  Transpose/1 -> Make UDP Packet/5(UDP Data)
  pktData/1 -> Transpose/1, Send_port_1002/1
  pktSize/1 -> DTC/1, Send_port_1002/2

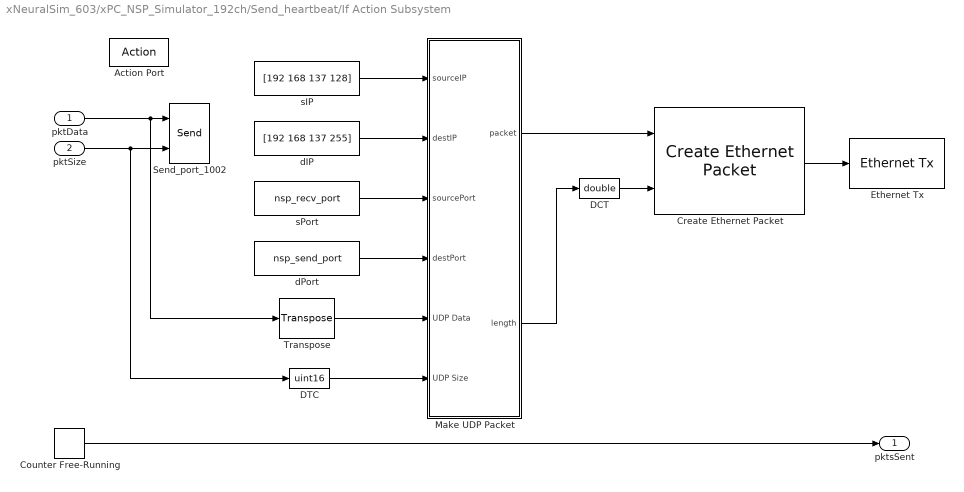
== system xNeuralSim_603/xPC_NSP_Simulator_192ch/Send_heartbeat/If Action Subsystem ==
  pktData : Inport
  pktSize : Inport  Port=2
  Action Port : ActionPort  ActionType=then
  Counter Free-Running : simulink/Sources/Counter Free-Running  NumBits=32  tsamp=-1
  Create Ethernet Packet : xpcethernetlib/Create Ethernet Packet   DstMac=macaddr('ff:ff:ff:ff:ff:ff')  EtherType=hex2dec('0800')
  DCT : DataTypeConversion  OutDataTypeStr=double
  DTC : DataTypeConversion  OutDataTypeStr=uint16
  Ethernet Tx : xpcethernetlib/Ethernet Tx   ID=2  SampleTime=-1
  Make UDP Packet : Subsystem
  Send_port_1002 : xpcrtudplib/Send   Send1=192.168.137.255  Send2=nsp_send_port  Send3=nsp_recv_port  Send4=-1
  Transpose : dspmtrx3/Transpose  Hermitian=off  overflowFlag=off
  dIP : Constant  Value=[192 168 137 255]  OutDataTypeStr=uint8
  dPort : Constant  Value=nsp_send_port  OutDataTypeStr=uint16
  sIP : Constant  Value=[192 168 137 128]  OutDataTypeStr=uint8
  sPort : Constant  Value=nsp_recv_port  OutDataTypeStr=uint16
  pktsSent : Outport  InitialOutput=0
  wires:
  Counter Free-Running/1 -> pktsSent/1
  DTC/1 -> Make UDP Packet/6(UDP Size)
  Make UDP Packet/2(length) -> DCT/1
  DCT/1 -> Create Ethernet Packet/2
  Make UDP Packet/1(packet) -> Create Ethernet Packet/1
  sPort/1 -> Make UDP Packet/3(sourcePort)
  Create Ethernet Packet/1 -> Ethernet Tx/1
  sIP/1 -> Make UDP Packet/1(sourceIP)
  dIP/1 -> Make UDP Packet/2(destIP)
  dPort/1 -> Make UDP Packet/4(destPort)
  Transpose/1 -> Make UDP Packet/5(UDP Data)
  pktData/1 -> Transpose/1, Send_port_1002/1
  pktSize/1 -> DTC/1, Send_port_1002/2

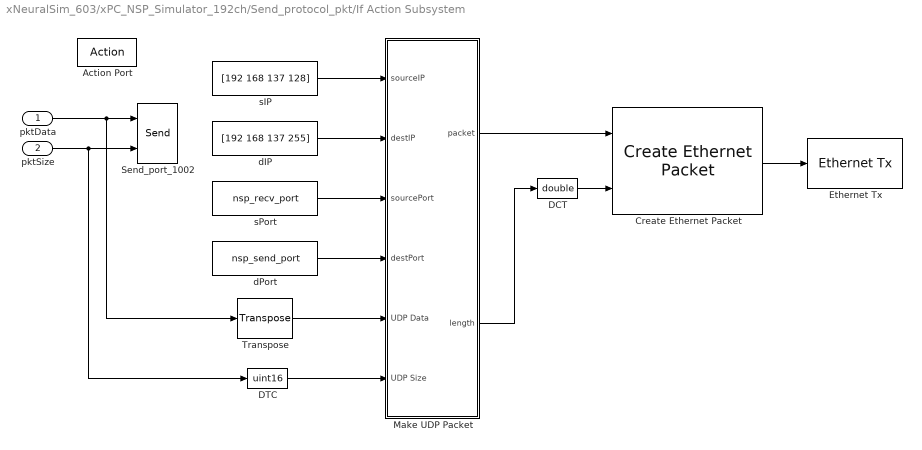
== system xNeuralSim_603/xPC_NSP_Simulator_192ch/Send_protocol_pkt/If Action Subsystem ==
  pktData : Inport
  pktSize : Inport  Port=2
  Action Port : ActionPort  ActionType=then
  Create Ethernet Packet : xpcethernetlib/Create Ethernet Packet   DstMac=macaddr('ff:ff:ff:ff:ff:ff')  EtherType=hex2dec('0800')
  DCT : DataTypeConversion  OutDataTypeStr=double
  DTC : DataTypeConversion  OutDataTypeStr=uint16
  Ethernet Tx : xpcethernetlib/Ethernet Tx   ID=2  SampleTime=-1
  Make UDP Packet : Subsystem
  Send_port_1002 : xpcrtudplib/Send   Send1=192.168.137.255  Send2=nsp_send_port  Send3=nsp_recv_port  Send4=-1
  Transpose : dspmtrx3/Transpose  Hermitian=off  overflowFlag=off
  dIP : Constant  Value=[192 168 137 255]  OutDataTypeStr=uint8
  dPort : Constant  Value=nsp_send_port  OutDataTypeStr=uint16
  sIP : Constant  Value=[192 168 137 128]  OutDataTypeStr=uint8
  sPort : Constant  Value=nsp_recv_port  OutDataTypeStr=uint16
  wires:
  DTC/1 -> Make UDP Packet/6(UDP Size)
  Make UDP Packet/2(length) -> DCT/1
  DCT/1 -> Create Ethernet Packet/2
  Make UDP Packet/1(packet) -> Create Ethernet Packet/1
  sPort/1 -> Make UDP Packet/3(sourcePort)
  Create Ethernet Packet/1 -> Ethernet Tx/1
  sIP/1 -> Make UDP Packet/1(sourceIP)
  dIP/1 -> Make UDP Packet/2(destIP)
  dPort/1 -> Make UDP Packet/4(destPort)
  Transpose/1 -> Make UDP Packet/5(UDP Data)
  pktData/1 -> Transpose/1, Send_port_1002/1
  pktSize/1 -> DTC/1, Send_port_1002/2

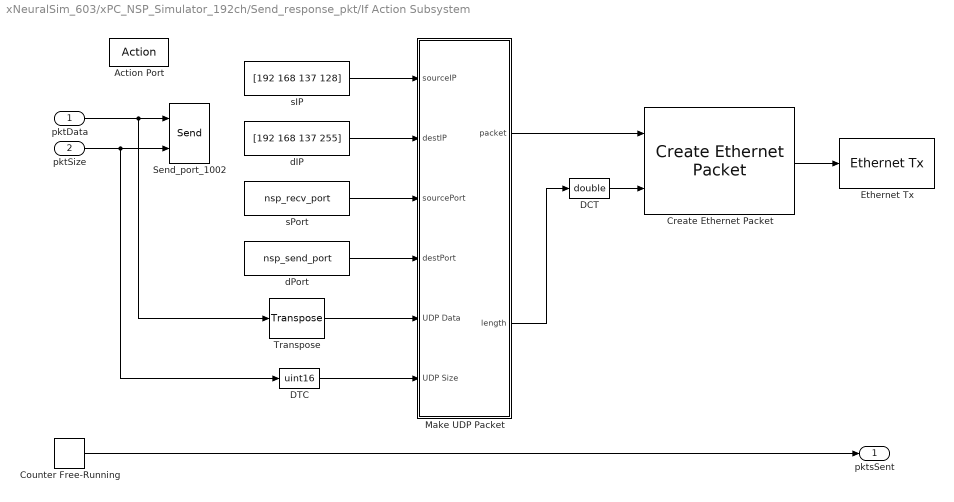
== system xNeuralSim_603/xPC_NSP_Simulator_192ch/Send_response_pkt/If Action Subsystem ==
  pktData : Inport
  pktSize : Inport  Port=2
  Action Port : ActionPort  ActionType=then
  Counter Free-Running : simulink/Sources/Counter Free-Running  NumBits=32  tsamp=-1
  Create Ethernet Packet : xpcethernetlib/Create Ethernet Packet   DstMac=macaddr('ff:ff:ff:ff:ff:ff')  EtherType=hex2dec('0800')
  DCT : DataTypeConversion  OutDataTypeStr=double
  DTC : DataTypeConversion  OutDataTypeStr=uint16
  Ethernet Tx : xpcethernetlib/Ethernet Tx   ID=2  SampleTime=-1
  Make UDP Packet : Subsystem
  Send_port_1002 : xpcrtudplib/Send   Send1=192.168.137.255  Send2=nsp_send_port  Send3=nsp_recv_port  Send4=-1
  Transpose : dspmtrx3/Transpose  Hermitian=off  overflowFlag=off
  dIP : Constant  Value=[192 168 137 255]  OutDataTypeStr=uint8
  dPort : Constant  Value=nsp_send_port  OutDataTypeStr=uint16
  sIP : Constant  Value=[192 168 137 128]  OutDataTypeStr=uint8
  sPort : Constant  Value=nsp_recv_port  OutDataTypeStr=uint16
  pktsSent : Outport  InitialOutput=0
  wires:
  Counter Free-Running/1 -> pktsSent/1
  DTC/1 -> Make UDP Packet/6(UDP Size)
  Make UDP Packet/2(length) -> DCT/1
  DCT/1 -> Create Ethernet Packet/2
  Make UDP Packet/1(packet) -> Create Ethernet Packet/1
  sPort/1 -> Make UDP Packet/3(sourcePort)
  Create Ethernet Packet/1 -> Ethernet Tx/1
  sIP/1 -> Make UDP Packet/1(sourceIP)
  dIP/1 -> Make UDP Packet/2(destIP)
  dPort/1 -> Make UDP Packet/4(destPort)
  Transpose/1 -> Make UDP Packet/5(UDP Data)
  pktData/1 -> Transpose/1, Send_port_1002/1
  pktSize/1 -> DTC/1, Send_port_1002/2

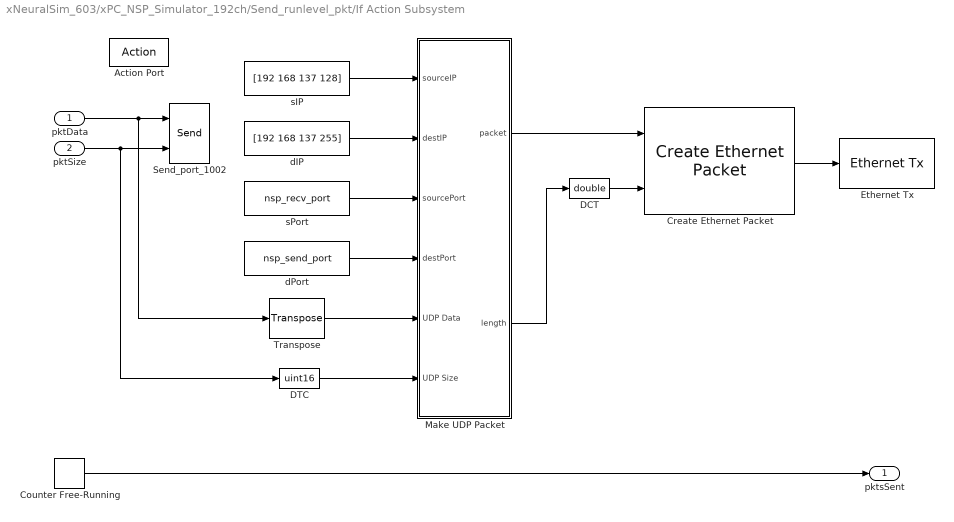
== system xNeuralSim_603/xPC_NSP_Simulator_192ch/Send_runlevel_pkt/If Action Subsystem ==
  pktData : Inport
  pktSize : Inport  Port=2
  Action Port : ActionPort  ActionType=then
  Counter Free-Running : simulink/Sources/Counter Free-Running  NumBits=32  tsamp=-1
  Create Ethernet Packet : xpcethernetlib/Create Ethernet Packet   DstMac=macaddr('ff:ff:ff:ff:ff:ff')  EtherType=hex2dec('0800')
  DCT : DataTypeConversion  OutDataTypeStr=double
  DTC : DataTypeConversion  OutDataTypeStr=uint16
  Ethernet Tx : xpcethernetlib/Ethernet Tx   ID=2  SampleTime=-1
  Make UDP Packet : Subsystem
  Send_port_1002 : xpcrtudplib/Send   Send1=192.168.137.255  Send2=nsp_send_port  Send3=nsp_recv_port  Send4=-1
  Transpose : dspmtrx3/Transpose  Hermitian=off  overflowFlag=off
  dIP : Constant  Value=[192 168 137 255]  OutDataTypeStr=uint8
  dPort : Constant  Value=nsp_send_port  OutDataTypeStr=uint16
  sIP : Constant  Value=[192 168 137 128]  OutDataTypeStr=uint8
  sPort : Constant  Value=nsp_recv_port  OutDataTypeStr=uint16
  pktsSent : Outport  InitialOutput=0
  wires:
  Counter Free-Running/1 -> pktsSent/1
  DTC/1 -> Make UDP Packet/6(UDP Size)
  Make UDP Packet/2(length) -> DCT/1
  DCT/1 -> Create Ethernet Packet/2
  Make UDP Packet/1(packet) -> Create Ethernet Packet/1
  sPort/1 -> Make UDP Packet/3(sourcePort)
  Create Ethernet Packet/1 -> Ethernet Tx/1
  sIP/1 -> Make UDP Packet/1(sourceIP)
  dIP/1 -> Make UDP Packet/2(destIP)
  dPort/1 -> Make UDP Packet/4(destPort)
  Transpose/1 -> Make UDP Packet/5(UDP Data)
  pktData/1 -> Transpose/1, Send_port_1002/1
  pktSize/1 -> DTC/1, Send_port_1002/2

== system xNeuralSim_603/xPC_NSP_Simulator_192ch/Spike_data_sender_NSP1/Send_sample_pkt ==
  pktData : Inport
  pktSize : Inport  Port=2
  cbPkts : Inport  Port=3
  If : If  ShowElse=off
  If Action Subsystem : Subsystem  TreatAsAtomicUnit=on
  pktsSent : Outport
  wires:
  pktData/1 -> If Action Subsystem/1(pktData)
  If/1 -> If Action Subsystem/Action
  pktSize/1 -> If Action Subsystem/2(pktSize), If/1
  If Action Subsystem/1(pktsSent) -> pktsSent/1
  cbPkts/1 -> If Action Subsystem/3(cbPkts)

== system xNeuralSim_603/xPC_NSP_Simulator_192ch/Spike_data_sender_NSP2/Send_sample_pkt ==
  pktData : Inport
  pktSize : Inport  Port=2
  cbPkts : Inport  Port=3
  If : If  ShowElse=off
  If Action Subsystem : Subsystem  TreatAsAtomicUnit=on
  pktsSent : Outport
  wires:
  pktData/1 -> If Action Subsystem/1(pktData)
  If/1 -> If Action Subsystem/Action
  pktSize/1 -> If Action Subsystem/2(pktSize), If/1
  If Action Subsystem/1(pktsSent) -> pktsSent/1
  cbPkts/1 -> If Action Subsystem/3(cbPkts)

== system xNeuralSim_603/xPC_NSP_Simulator_192ch/Sample_data_sender_NSP1/Send_sample_pkt/If Action Subsystem ==
  pktData : Inport
  pktSize : Inport  Port=2
  cbPkts1 : Inport  Port=3
  Action Port : ActionPort  ActionType=then
  Add : Sum  AccumDataTypeStr=uint32  OutDataTypeStr=uint32
  Send_port_1002 : Subsystem  mask(send){Send1=192.168.137.255, Send2=nsp_send_port, Send3=nsp_recv_port, Send4=-1}
      mask prompts: Send1 "IP address to send to (255.255.255.255 for broadcast):"; Send2 "Remote IP port to send to:"; Send3 "Use the following local IP port (-1 for automatic assignment):"; Send4 "Sample time:"
      mask init:
      | Send1 = ipaddr(Send1);
      mask Help: helpview(fullfile(docroot, 'mapfiles', 'xpc.map'), 'RT_UDP_SEND')
      mask Display: disp('UDP\nSend')
  Unit Delay : UnitDelay  SampleTime=-1
  pktsSent1 : Outport  InitialOutput=0
  wires:
  Add/1 -> Unit Delay/1, pktsSent1/1
  Unit Delay/1 -> Add/2
  cbPkts1/1 -> Add/1
  pktData/1 -> Send_port_1002/1(In1)
  pktSize/1 -> Send_port_1002/2(In2)
